simulink model "dos"  (R2020a)
settings: Solver=VariableStepAuto  StartTime=0.0  StopTime=10.0  RelTol=1e-3
undefined symbols (not defined in the file): heaviside
settings Model: Creator=mluser  LastModifiedBy=mluser

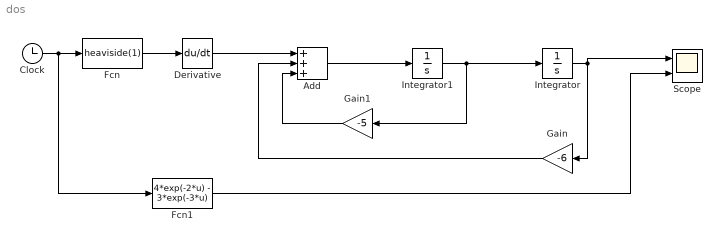
== system dos ==
  Add : Sum  Inputs=+++
  Clock : Clock
  Derivative : Derivative
  Fcn : Fcn  Expr=heaviside(1)
  Fcn1 : Fcn  Expr=4*exp(-2*u) - 3*exp(-3*u)
  Gain : Gain  Gain=-6
  Gain1 : Gain  Gain=-5
  Integrator : Integrator  InitialCondition=1
  Integrator1 : Integrator  InitialCondition=1
  Scope : Scope  NumInputPorts=2
  wires:
  Clock/1 -> Fcn1/1, Fcn/1
  Fcn/1 -> Derivative/1
  Derivative/1 -> Add/1
  Add/1 -> Integrator1/1
  Integrator1/1 -> Integrator/1, Gain1/1
  Gain1/1 -> Add/3
  Integrator/1 -> Scope/1, Gain/1
  Gain/1 -> Add/2
  Fcn1/1 -> Scope/2
